simulink model "RLC"  (Simulink 9.0)
settings: Solver=VariableStepAuto  StartTime=0.0  StopTime=4e-2  MaxStep=10^-6  RelTol=1e-3
values from neighbouring files (symbols this model uses):
  K1 = 1/L    (= 1000)    [lab1.m]
  K2 = 1/c    (= 1000)    [lab1.m]
  K3 = 1/(R*c)    (= 500)    [lab1.m]
settings Model: Creator=Charlene Shong  LastModifiedBy=Charlene Shong
settings DataIOCC: SaveFormat=Dataset
settings OptimizationCC: LifeSpan=auto
settings DebuggingCC: UnderspecifiedInitializationDetection=Simplified  MergeDetectMultiDrivingBlocksExec=error  SFUnexpectedBacktrackingDiag=error  SFNoUnconditionalDefaultTransitionDiag=error  SFExecutionAtInitializationDiag=warning
settings HardwareCC: ProdBitPerPointer=64  ProdBitPerSizeT=64  ProdBitPerPtrDiffT=64  ProdLargestAtomicFloat=Float  ProdIntDivRoundTo=Zero  ProdEndianess=LittleEndian  ProdWordSize=64  ProdHWDeviceType=Intel->x86-64 (Windows64)
settings ModelReferenceCC: PropagateSignalLabelsOutOfModel=on
settings CodeAppCC: StateflowObjectComments=off
settings GRTTargetCC: TargetLangStandard=C99 (ISO)
settings ConfigComp: CovMetricSettings=dwe  CovHtmlReporting=off  CovSaveCumulativeToWorkspaceVar=off  CovSaveSingleToWorkspaceVar=off  CovExternalEMLEnable=on

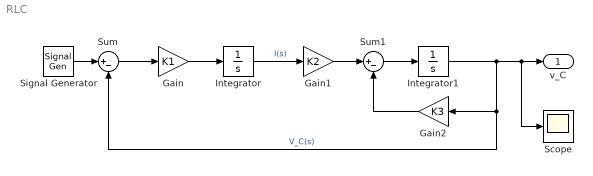
== system RLC ==
  Gain : Gain  Gain=K1
  Gain1 : Gain  Gain=K2
  Gain2 : Gain  Gain=K3
  Integrator : Integrator
  Integrator1 : Integrator  InitialCondition=1
  Scope : Scope
  Signal Generator : SignalGenerator  WaveForm=square  Frequency=25
  Sum : Sum  Inputs=|+-
  Sum1 : Sum  Inputs=|+-
  v_C : Outport
  wires:
  Sum/1 -> Gain/1
  Gain/1 -> Integrator/1
  Integrator/1 -> Gain1/1  "I(s)"
  Gain1/1 -> Sum1/1
  Sum1/1 -> Integrator1/1
  Integrator1/1 -> Scope/1, v_C/1, Gain2/1, Sum/2  "V_C(s)"
  Gain2/1 -> Sum1/2
  Signal Generator/1 -> Sum/1
